simulink model "QCar2_DetailedScenario-2025a"  (R2025a)
settings: Solver=ode2  StartTime=0.0  StopTime=inf  FixedStep=1/100  RelTol=1e-3  EnableMultiTasking=on
model workspace (MAT data in the model file):
  XY_OFFSET : Simulink.Parameter (value not decoded)
  camera_rate : Simulink.Parameter (value not decoded)
  depth_rate : Simulink.Parameter (value not decoded)
  path_to_pickup : Simulink.Parameter (value not decoded)
  path_to_pickup_tight : Simulink.Parameter (value not decoded)
symbols that are objects in the model workspace (value not decoded): camera_rate, depth_rate, path_to_pickup, XY_OFFSET
undefined symbols (not defined in the file or in its folder): gcbh, HIL, JPEG, Point, qc_get_step_size, Video3D, video_display_show
libraries: quarc_library x37, simulink x16
(part 3 of 3)

== matlab function QCar2_DetailedScenario-2025a/basicQCarIO/lidarLaneFollower ==
  data: dist input; v_out output; ang input; dt input; omega_out output; laneConf output; roadRisk output
% function [v_out, omega_out] = lidarLaneFollower(dist, ang, dt)
% %#codegen
% % dist, ang: 360x1
% % outputs: v_out (m/s), omega_out (rad/s)
% 
% % ---- Force shapes / scalars ----
% dist = dist(:);
% ang  = ang(:);
% dt   = double(dt(1));
% 
% % ---- Parameters you can tune quickly ----
% lane_half_width = 1.2;     % meters (half of drivable corridor; start ~1.0-1.5)
% look_deg        = 70;      % use ±look_deg to "see" boundaries
% minR = 0.15; maxR = 20.0;
% 
% Kp = 1.2;                  % steering from lateral error
% Kd = 0.15;                 % damping
% Kw = 0.6;                  % yaw-rate damping (stability)
% 
% omega_max = 0.9;           % rad/s
% v_min = 0.4;
% v_max = 1.5;
% 
% persistent e_prev
% if isempty(e_prev)
%     e_prev = 0;
% end
% 
% % ---- Filter invalid ranges ----
% valid = isfinite(dist) & isfinite(ang) & dist>minR & dist<maxR;
% 
% % If scan is garbage, stop
% if nnz(valid) < 50
%     v_out = 0.0;
%     omega_out = 0.0;
%     return;
% end
% 
% % ---- Grab points near left and right sides ----
% % We want distances around +look (left) and -look (right) relative to forward.
% look = look_deg*pi/180;
% 
% % Define angular windows (in radians)
% w = 12*pi/180;    % ±12 deg window
% 
% leftMask  = valid & (ang > ( look - w)) & (ang < ( look + w));
% rightMask = valid & (ang > (-look - w)) & (ang < (-look + w));
% 
% % Robust boundary distance: use median of projected lateral distances
% % Lateral distance approx: y = r*sin(theta)
% % Positive y = left side, negative y = right side.
% yl = dist(leftMask)  .* sin(ang(leftMask));
% yr = dist(rightMask) .* sin(ang(rightMask));  % negative values
% 
% % If one side missing, fall back to wall-following on the other side
% haveL = ~isempty(yl);
% haveR = ~isempty(yr);
% 
% if haveL
%     dL = median(yl);     % should be positive
% else
%     dL = lane_half_width;
% end
% 
% if haveR
%     dR = -median(yr);    % convert to positive distance
% else
%     dR = lane_half_width;
% end
% 
% % ---- Lateral centering error ----
% % If centered: dL ~= dR (depends), but for symmetric corridor you want dL == dR.
% e = (dL - dR);     % positive means too close to right -> steer right? (we’ll handle sign below)
% 
% % Derivative
% de = (e - e_prev) / max(dt, 1e-3);
% e_prev = e;
% 
% % ---- Estimate curvature demand from forward sector (optional) ----
% % A cheap proxy: if we see closer obstacles in front-left vs front-right, turn away.
% frontW = 25*pi/180;
% frontL = valid & (ang > 0) & (ang < frontW);
% frontR = valid & (ang < 0) & (ang > -frontW);
% 
% fL = median(dist(frontL));
% fR = median(dist(frontR));
% if ~isfinite(fL), fL = 10; end
% if ~isfinite(fR), fR = 10; end
% curv_hint = (fR - fL);  % if left is tighter (smaller fL), this becomes positive -> steer right
% 
% % ---- Steering law (omega) ----
% % Sign convention: if dL > dR, you’re closer to right -> steer left (positive omega)
% omega =  Kp*e + Kd*de + 0.15*curv_hint;
% omega = omega - Kw*0;   % (if you have yaw-rate gyro, subtract it here)
% 
% % Clamp
% if omega > omega_max, omega = omega_max; end
% if omega < -omega_max, omega = -omega_max; end
% 
% % ---- Speed scheduling: slower when turning more ----
% v = v_max * (1.0 - min(abs(omega)/omega_max, 1.0)*0.6);
% v = max(v_min, v);
% 
% % If we lost one boundary, slow down
% if ~(haveL && haveR)
%     v = min(v, 0.7);
% end
% 
% v_out = double(v);
% omega_out = double(omega);
% end
% function [v_out, omega_out] = lidarLaneFollower(dist, ang, dt)
% %#codegen
% % dist, ang: 360x1
% % outputs: v_out (m/s), omega_out (rad/s)
% 
% % ---- Force shapes / scalars ----
% dist = dist(:);
% ang  = ang(:);
% dt   = double(dt(1));
% 
% % ---- Parameters you can tune quickly ----
% lane_half_width = 1.2;     % meters (half of drivable corridor; start ~1.0-1.5)
% look_deg        = 70;      % use ±look_deg to "see" boundaries
% minR = 0.15; maxR = 20.0;
% 
% Kp = 1.2;                  % steering from lateral error
% Kd = 0.15;                 % damping
% Kw = 0.6;                  % yaw-rate damping (stability)
% 
% omega_max = 0.9;           % rad/s
% v_min = 0.4;
% v_max = 1.5;
% 
% persistent e_prev
% if isempty(e_prev)
%     e_prev = 0;
% end
% 
% % ---- Filter invalid ranges ----
% valid = isfinite(dist) & isfinite(ang) & dist>minR & dist<maxR;
% 
% % If scan is garbage, stop
% if nnz(valid) < 50
%     v_out = 0.0;
%     omega_out = 0.0;
%     return;
% end
% 
% % ---- Grab points near left and right sides ----
% % We want distances around +look (left) and -look (right) relative to forward.
% look = look_deg*pi/180;
% 
% % Define angular windows (in radians)
% w = 12*pi/180;    % ±12 deg window
% 
% leftMask  = valid & (ang > ( look - w)) & (ang < ( look + w));
% rightMask = valid & (ang > (-look - w)) & (ang < (-look + w));
% 
% % Robust boundary distance: use median of projected lateral distances
% % Lateral distance approx: y = r*sin(theta)
% % Positive y = left side, negative y = right side.
% yl = dist(leftMask)  .* sin(ang(leftMask));
% yr = dist(rightMask) .* sin(ang(rightMask));  % negative values
% 
% % If one side missing, fall back to wall-following on the other side
% haveL = ~isempty(yl);
% haveR = ~isempty(yr);
% 
% if haveL
%     dL = median(yl);     % should be positive
% else
%     dL = lane_half_width;
% end
% 
% if haveR
%     dR = -median(yr);    % convert to positive distance
% else
%     dR = lane_half_width;
% end
% 
% % ---- Lateral centering error ----
% % If centered: dL ~= dR (depends), but for symmetric corridor you want dL == dR.
% e = (dL - dR);     % positive means too close to right -> steer right? (we’ll handle sign below)
% 
% % Derivative
% de = (e - e_prev) / max(dt, 1e-3);
% e_prev = e;
% 
% % ---- Estimate curvature demand from forward sector (optional) ----
% % A cheap proxy: if we see closer obstacles in front-left vs front-right, turn away.
% frontW = 25*pi/180;
% frontL = valid & (ang > 0) & (ang < frontW);
% frontR = valid & (ang < 0) & (ang > -frontW);
% 
% fL = median(dist(frontL));
% fR = median(dist(frontR));
% if ~isfinite(fL), fL = 10; end
% if ~isfinite(fR), fR = 10; end
% curv_hint = (fR - fL);  % if left is tighter (smaller fL), this becomes positive -> steer right
% 
% % ---- Steering law (omega) ----
% % Sign convention: if dL > dR, you’re closer to right -> steer left (positive omega)
% omega =  Kp*e + Kd*de + 0.15*curv_hint;
% omega = omega - Kw*0;   % (if you have yaw-rate gyro, subtract it here)
% 
% % Clamp
% if omega > omega_max, omega = omega_max; end
% if omega < -omega_max, omega = -omega_max; end
% 
% % ---- Speed scheduling: slower when turning more ----
% v = v_max * (1.0 - min(abs(omega)/omega_max, 1.0)*0.6);
% v = max(v_min, v);
% 
% % If we lost one boundary, slow down
% if ~(haveL && haveR)
%     v = min(v, 0.7);
% end
% 
% v_out = double(v);
% omega_out = double(omega);
% end
function [v_out, omega_out, laneConf, roadRisk] = lidarLaneFollower(dist, ang, dt)
%#codegen
% Robust corridor follower from 2D LiDAR.
% dist, ang: 360x1 (ang=0 forward, + left)
% outputs: v_out (m/s), omega_out (rad/s), laneConf [0..1], roadRisk [0..1]

dist = dist(:);
ang  = ang(:);
dt   = double(dt(1));
if dt <= 0, dt = 0.02; end

% ---------- Tunables ----------
minR = 0.15; maxR = 20.0;

% Side sectors used to detect corridor boundaries (deg)
left_deg  = [20  115];
right_deg = [-115 -20];

x_min = 0.35;      % ignore very close points
x_look = 1.20;     % lookahead for center measurement

% corridor half-width guess for one-side fallback
lane_half_guess = 1.25;

% Controller gains (stable defaults)
k_psi = 1.6;          % heading correction
k_y   = 1.2;          % lateral correction gain
k_y_atan = 1.6;       % atan sensitivity

omega_max = 0.9;
v_min = 0.45;
v_max = 1.4;

% Minimum points
minPtsSide = 22;
minTotalValid = 80;

% Residual thresholds (meters) for fit quality
res_good = 0.10;
res_bad  = 0.28;

% risk thresholds (meters)
e_warn   = 0.40;
e_freeze = 1.10;

% Smoothing (time-constant style)
tau_omega = 0.18;     % sec
tau_center = 0.25;    % sec
tau_heading = 0.25;   % sec
% ----------------------------

% persistent filters / memory
persistent omega_filt ycen_filt psiref_filt initialized
if isempty(initialized)
    initialized = true;
    omega_filt  = 0.0;
    ycen_filt   = 0.0;
    psiref_filt = 0.0;
end

% ---------- Validate scan ----------
valid = isfinite(dist) & isfinite(ang) & dist > minR & dist < maxR;
if nnz(valid) < minTotalValid
    v_out = 0.0;
    omega_out = 0.0;
    laneConf = 0.0;
    roadRisk = 1.0;
    return;
end

% ---------- Convert to Cartesian ----------
r  = dist(valid);
th = ang(valid);
x  = r .* cos(th);
y  = r .* sin(th);
deg = th * (180/pi);

% ---------- Select left/right wall points ----------
Lmask = (deg >= left_deg(1))  & (deg <= left_deg(2))  & (x > x_min);
Rmask = (deg >= right_deg(1)) & (deg <= right_deg(2)) & (x > x_min);

xL = x(Lmask); yL = y(Lmask);
xR = x(Rmask); yR = y(Rmask);

nL = numel(xL);
nR = numel(xR);

haveL = (nL >= minPtsSide);
haveR = (nR >= minPtsSide);

% ---------- Fit left/right lines with trimming ----------
% returns: m,b,res (median absolute residual)
mL = 0; bL = 0; resL = 1e9;
mR = 0; bR = 0; resR = 1e9;

if haveL
    [mL, bL, resL] = fitLineTrimmed(xL, yL);
end
if haveR
    [mR, bR, resR] = fitLineTrimmed(xR, yR);
end

% Decide if each side is reliable by residual
okL = haveL && isfinite(mL) && isfinite(bL) && (resL < res_bad);
okR = haveR && isfinite(mR) && isfinite(bR) && (resR < res_bad);

haveBoth = okL && okR;

% ---------- Compute corridor center + heading ----------
y_center = ycen_filt;     % default to memory
psi_ref  = psiref_filt;

if haveBoth
    % evaluate both lines at x_look
    yL_at = mL*x_look + bL;
    yR_at = mR*x_look + bR;
    y_center = 0.5*(yL_at + yR_at);

    % heading from average slope
    mC = 0.5*(mL + mR);
    psi_ref = atan(mC);
elseif okL
    % follow left wall: center is left wall minus half width
    yL_at = mL*x_look + bL;
    y_center = yL_at - lane_half_guess;
    psi_ref = atan(mL);
elseif okR
    % follow right wall: center is right wall plus half width
    yR_at = mR*x_look + bR;
    y_center = yR_at + lane_half_guess;
    psi_ref = atan(mR);
else
    % nothing reliable: keep filtered memory (don’t snap)
    y_center = ycen_filt;
    psi_ref  = psiref_filt;
end

% ---------- Low-pass filter center and heading ----------
aC = dt / max(tau_center + dt, 1e-6);
aH = dt / max(tau_heading + dt, 1e-6);
ycen_filt   = (1-aC)*ycen_filt   + aC*y_center;
psiref_filt = (1-aH)*psiref_filt + aH*psi_ref;

y_center = ycen_filt;
psi_ref  = psiref_filt;

% ---------- Confidence (0..1) ----------
% Count-based confidence
cL = min(1.0, double(nL)/double(2*minPtsSide));
cR = min(1.0, double(nR)/double(2*minPtsSide));
cCount = min(cL, cR);

% Residual-based confidence
qL = qualityFromResidual(resL, res_good, res_bad);
qR = qualityFromResidual(resR, res_good, res_bad);

if haveBoth
    cFit = min(qL, qR);
else
    % one-side fallback is inherently less confident
    cFit = 0.4 * max(qL, qR);
    cCount = 0.6 * max(cL, cR);
end

laneConf = min(1.0, max(0.0, 0.6*cFit + 0.4*cCount));

% ---------- Road risk (0..1) ----------
absE = abs(y_center);

if absE <= e_warn
    risk_e = 0.0;
elseif absE >= e_freeze
    risk_e = 1.0;
else
    risk_e = (absE - e_warn) / (e_freeze - e_warn);
end

risk_conf = 1.0 - laneConf;
roadRisk = max(risk_e, risk_conf);

% ---------- Controller (omega) ----------
psi_err = wrapToPi(psi_ref);

% bounded lateral term (Stanley-ish)
v_guess = v_max;
lat_term = atan2(k_y_atan * y_center, (v_guess + 0.25));

omega = k_psi*psi_err + k_y*lat_term;

omega = max(-omega_max, min(omega_max, omega));

% omega low-pass
aW = dt / max(tau_omega + dt, 1e-6);
omega_filt = (1-aW)*omega_filt + aW*omega;
omega = omega_filt;

% ---------- Speed scheduling ----------
turnSlow = 1.0 - 0.65*min(abs(omega)/omega_max, 1.0);
confSlow = 0.35 + 0.65*laneConf;

v = v_max * turnSlow * confSlow;
v = max(v_min, min(v_max, v));

% If very risky or not confident: slow more
if roadRisk > 0.85
    v = min(v, 0.55);
elseif laneConf < 0.25
    v = min(v, 0.70);
end

v_out = double(v);
omega_out = double(omega);
laneConf = double(laneConf);
roadRisk = double(roadRisk);
end

% ===== helper functions =====

function q = qualityFromResidual(res, good, bad)
%#codegen
if ~isfinite(res)
    q = 0.0;
    return;
end
if res <= good
    q = 1.0;
elseif res >= bad
    q = 0.0;
else
    q = (bad - res) / (bad - good);
end
end

function [m, b, medAbsRes] = fitLineTrimmed(x, y)
%#codegen
% Two-pass trimmed least squares fit for y = m x + b

x = double(x(:));
y = double(y(:));
n = numel(x);

% default
m = NaN; b = NaN; medAbsRes = 1e9;
if n < 10
    return;
end

% pass 1
[m1, b1] = fitLineLS(x, y);
if ~isfinite(m1) || ~isfinite(b1)
    return;
end

r = y - (m1*x + b1);
ar = abs(r);

% keep best fraction
frac = 0.70;
k = max(10, floor(frac*n));

% find threshold by partial selection (simple sort is OK at 360 points)
ar_sorted = sort(ar);
th = ar_sorted(k);

keep = (ar <= th);
x2 = x(keep);
y2 = y(keep);

% pass 2
[m2, b2] = fitLineLS(x2, y2);
if ~isfinite(m2) || ~isfinite(b2)
    m = m1; b = b1;
else
    m = m2; b = b2;
end

% median abs residual as quality metric
r2 = y - (m*x + b);
medAbsRes = median(abs(r2));
end

function [m, b] = fitLineLS(x, y)
%#codegen
n = numel(x);
m = NaN; b = NaN;
if n < 2
    return;
end

sx  = sum(x);
sy  = sum(y);
sxx = sum(x.*x);
sxy = sum(x.*y);

den = (n*sxx - sx*sx);
if abs(den) < 1e-9
    return;
end

m = (n*sxy - sx*sy) / den;
b = (sy - m*sx) / n;
end

function a = wrapToPi(x)
%#codegen
a = mod(x+pi, 2*pi) - pi;
end

== matlab function QCar2_DetailedScenario-2025a/CommandFusion ==
  data: v_wp input; v_cmd output; omega_wp input; v_vis input; omega_vis input; visValid input; v_lane input; omega_lane input; laneConf input; roadRisk input; omega_cmd output; alpha_safety output; alpha_vis output
function [v_cmd, omega_cmd, alpha_safety, alpha_vis] = CommandFusion( ...
    v_wp, omega_wp, v_vis, omega_vis, visValid, v_lane, omega_lane, laneConf, roadRisk)
%#codegen

v_wp      = double(v_wp(1));     omega_wp   = double(omega_wp(1));
v_vis     = double(v_vis(1));    omega_vis  = double(omega_vis(1));
visValid  = double(visValid(1));
v_lane    = double(v_lane(1));   omega_lane = double(omega_lane(1));
laneConf  = double(laneConf(1)); roadRisk   = double(roadRisk(1));

visValid = min(max(visValid,0),1);
laneConf = min(max(laneConf,0),1);
roadRisk = min(max(roadRisk,0),1);

% ---- (A) Intent steering: waypoint + vision
% Ignore vision speed if it's not meaningful
if v_vis <= 0.05
    v_vis = v_wp;
end

% Vision helps, but don’t let it dominate unless it's valid
alpha_vis = 0.7 * visValid;    % was 0.85 (too aggressive)
omega_intent = (1-alpha_vis)*omega_wp + alpha_vis*omega_vis;

% ---- (B) Safety takeover: ONLY when lane is confident and risk is real
% Make alpha_safety ~0 unless roadRisk is high
risk_on  = 0.35;   % start takeover
risk_full= 0.85;   % full takeover

if roadRisk <= risk_on
    a = 0.0;
elseif roadRisk >= risk_full
    a = 1.0;
else
    a = (roadRisk - risk_on) / (risk_full - risk_on);
end

alpha_safety = a * laneConf;   % no confidence => no takeover

% ---- (C) Final omega
omega_cmd = (1-alpha_safety)*omega_intent + alpha_safety*omega_lane;

% ---- (D) Speed: use waypoint speed, clamp only if laneConf is good
v_intent = max(v_wp, 0.0);

if laneConf > 0.4
    v_cmd = min(v_intent, max(v_lane, 0.0));
else
    v_cmd = v_intent;
end

% ---- clamps
omega_max = 0.9;
omega_cmd = max(-omega_max, min(omega_max, omega_cmd));
end

== matlab function QCar2_DetailedScenario-2025a/obstacleDetection/Draw Lines Module ==
  data: img_in input; img_out output; pts input; color input
function img_out = drawLines(img_in, pts, color)

% Draw lines connecting the points using the provided color

% Inputs:
% img_in    : Input RGB Image (size = m by n)
% pts       : p x-y pairs of points (px) where markers are to be drawn
% color     : 1x3 matrix of RGB color values for each marker

% Outputs:
% img_out   : Output RGB Image with the markers drawn in (size = m by n)

%% Initialization
if size(img_in, 3) == 3
    img_out = img_in;
elseif size(img_in, 3) == 1
    img_out = cat(3, img_in, img_in, img_in);
end

[p, ~] = size(pts); % determine the number of points
%% Draw the lines
    for i = 1:p-1
        % determine the max(rows_difference, col_difference) between two
        % points
        itr = max(abs(pts(i,1) - pts(i+1,1)), abs(pts(i,2) - pts(i+1,2)));
        
        % generate linear spaces of row and col values between the pts
        row_vec = ceil(linspace(pts(i,1), pts(i+1,1), itr));
        col_vec = ceil(linspace(pts(i,2), pts(i+1,2), itr));
        
        % iterate through the values and shade them right

        for j = 1:itr
            img_out(row_vec(j), col_vec(j),1) = color(1);
            img_out(row_vec(j), col_vec(j),2) = color(2);
            img_out(row_vec(j), col_vec(j),3) = color(3);
        end
    end
end

== matlab function QCar2_DetailedScenario-2025a/steeringCalculation/Find slope and intercept ==
  data: Binary input; m output; b output; laneSelector input; imageSize input
function [m, b] = linearPolyFit(Binary, laneSelector, imageSize)

% find the shape of the incoming image
[ROW, ~] = size(Binary);

% find row, col pairs of points where pixel value is bright
[rows, cols] = find(Binary(ROW - imageSize(1) + 1:end, :) > 0);

% x is coloumns, y is max_row - rows
if laneSelector
    x = imageSize(2) - cols;
else
    x = cols;
end

y = imageSize(1) - rows;

% fit a linear polynomial to the points and grab slope, intercept
% result = polyfit(x(idx), y(idx), 1);
result = polyfit(x, y, 1);
m = result(1); 
b = result(2);

== stateflow chart QCar2_DetailedScenario-2025a/TaxiHubSupervisor  ==
  state INIT
    entry:
    arm = false;
    mode = false;
  state ARMING
    entry:
    arm = true;
    mode = false;
  state WaypointFollowing
    entry:
    arm = true;
    mode = false;
    during:
    arm = true;
    mode = false;
  state SEARCH_LANE
    entry:
    arm = true;
    mode = false;
    during:
  state LANE_FOLLOW
    entry:
    arm = true;
    mode = true;
    during:
  (default) -> INIT
  INIT -> ARMING : after(t_init, sec)
  ARMING -> WaypointFollowing : after(t_arm, sec)
  WaypointFollowing -> SEARCH_LANE : [wp_reached_in > 0.5]
  SEARCH_LANE -> LANE_FOLLOW : [laneStable || after(1,sec)]
  data: mode output boolean size=1; arm output boolean size=1; laneStable input boolean size=1; t_init local double size=1 =0.5; t_arm local double size=1 =0.5; wp_reached_in input double size=1
